simulink model "Simulink_lab3"  (R2020a)
settings: Solver=VariableStepAuto  StartTime=0.0  StopTime=25  RelTol=1e-3
libraries: cstblocks x3
settings Model: Creator=X1  LastModifiedBy=me-clab2
settings DebuggingCC: UnconnectedInputMsg=none  UnconnectedOutputMsg=none  UnconnectedLineMsg=none  SFMachineParentedDataDiag=error
settings ModelReferenceCC: EnableRefExpFcnMdlSchedulingChecks=off
settings RTWCC: Description=Generic Real-Time Target

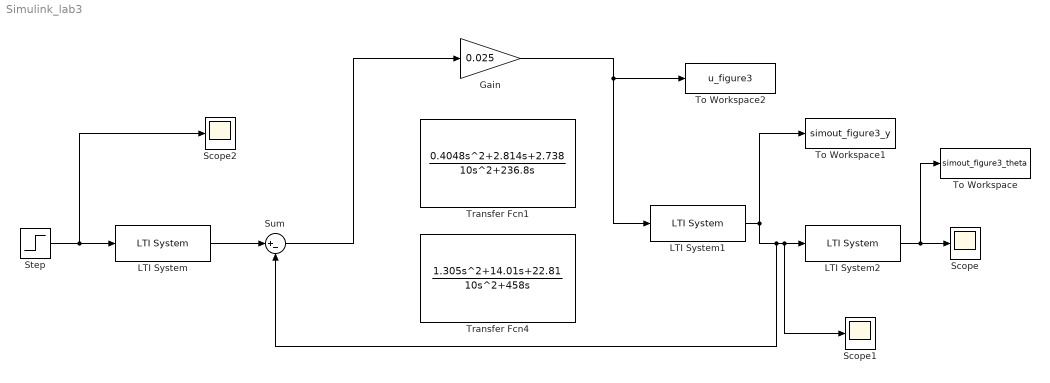
== system Simulink_lab3 ==
  Gain : Gain  Gain=0.025
  LTI System : cstblocks/LTI System  sys=F  IC=[]
  LTI System1 : cstblocks/LTI System  sys=Py  IC=[]
  LTI System2 : cstblocks/LTI System  sys=P_theta  IC=[]
  Scope : Scope
  Scope1 : Scope
  Scope2 : Scope
  Step : Step  SampleTime=0
  Sum : Sum  Inputs=|+-
  To Workspace : ToWorkspace  VariableName=simout_figure3_theta  SaveFormat=Structure With Time  SampleTime=-1
  To Workspace1 : ToWorkspace  VariableName=simout_figure3_y  SaveFormat=Structure With Time  SampleTime=-1
  To Workspace2 : ToWorkspace  VariableName=u_figure3  SaveFormat=Timeseries  SampleTime=-1
  Transfer Fcn1 : TransferFcn  Numerator=[0.4048 2.814 2.738]  Denominator=[10 236.8 0]
  Transfer Fcn4 : TransferFcn  Numerator=[1.305 14.01 22.81]  Denominator=[10 458 0]
  wires:
  LTI System/1 -> Sum/1
  LTI System1/1 -> Sum/2, Scope1/1, LTI System2/1, To Workspace1/1
  LTI System2/1 -> To Workspace/1, Scope/1
  Step/1 -> Scope2/1, LTI System/1
  Sum/1 -> Gain/1
  Gain/1 -> LTI System1/1, To Workspace2/1
